simulink model "bit32aluhdl"  (R2020a)
settings: Solver=FixedStepDiscrete  StartTime=0.0  StopTime=10.0  RelTol=1e-3
(part 1 of 66)
settings Model: DataTypeOverride=Off  Creator=kishan  LastModifiedBy=kishan
settings DataIOCC: LimitDataPoints=on  SaveOutput=off  SaveTime=off
settings OptimizationCC: BlockReduction=off  ConditionallyExecuteInputs=off  DefaultParameterBehavior=Inlined  ExpressionDepthLimit=2147483647  InitFltsAndDblsToZero=on  LifeSpan=inf
settings DebuggingCC: AlgebraicLoopMsg=error  UnderspecifiedInitializationDetection=Classic  MergeDetectMultiDrivingBlocksExec=none  SingleTaskRateTransMsg=error  FcnCallInpInsideContextMsg=warning  AllowSymbolicDim=off  StateNameClashWarn=warning  StrictBusMsg=ErrorOnBusTreatedAsVector  SFUnexpectedBacktrackingDiag=warning  SFNoUnconditionalDefaultTransitionDiag=warning  SFExecutionAtInitializationDiag=none  ArithmeticOperatorsInVariantConditions=warning
settings HardwareCC: ProdBitPerPointer=32  ProdBitPerSizeT=32  ProdBitPerPtrDiffT=32  ProdLargestAtomicFloat=None  ProdIntDivRoundTo=Undefined  ProdEndianess=Unspecified  ProdWordSize=32  ProdHWDeviceType=ASIC/FPGA->ASIC/FPGA  ProdEqTarget=off
settings SFSimCC: SimUseLocalCustomCode=off  SimParseCustomCode=off  CustomCodeUndefinedFunction=UseInterfaceOnly
settings RTWCC: RTWUseLocalCustomCode=off
settings CodeAppCC: StateflowObjectComments=on
settings GRTTargetCC: TargetLangStandard=C89/C90 (ANSI)  CombineOutputUpdateFcns=off  GRTInterface=on
settings ConfigComp: CovScope=ReferencedModels  CovMetricSettings=dw  CovHtmlReporting=on  CovSaveCumulativeToWorkspaceVar=on  CovSaveSingleToWorkspaceVar=on  CovExternalEMLEnable=off  CovSFcnEnable=off

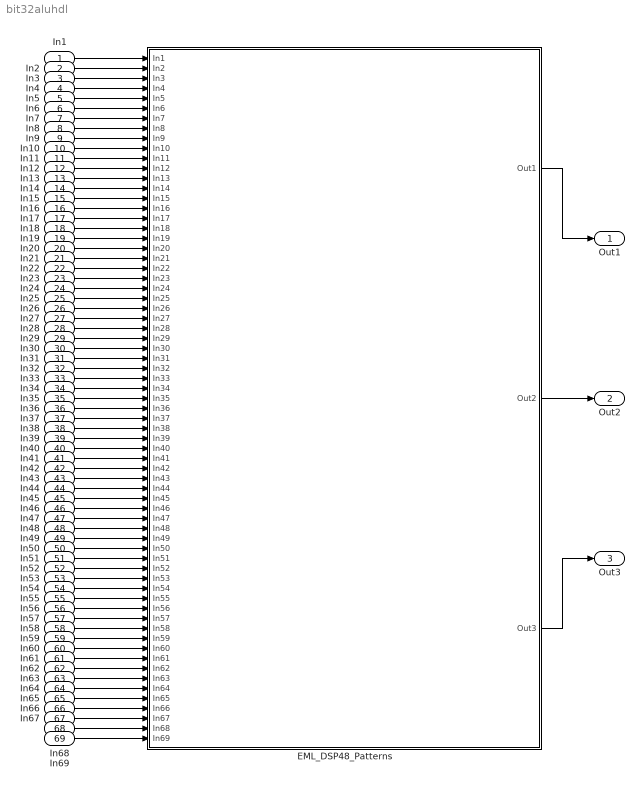
== system bit32aluhdl ==
  In1 : Inport
  In2 : Inport  Port=2
  In3 : Inport  Port=3
  In4 : Inport  Port=4
  In5 : Inport  Port=5
  In6 : Inport  Port=6
  In7 : Inport  Port=7
  In8 : Inport  Port=8
  In9 : Inport  Port=9
  In10 : Inport  Port=10
  In11 : Inport  Port=11
  In12 : Inport  Port=12
  In13 : Inport  Port=13
  In14 : Inport  Port=14
  In15 : Inport  Port=15
  In16 : Inport  Port=16
  In17 : Inport  Port=17
  In18 : Inport  Port=18
  In19 : Inport  Port=19
  In20 : Inport  Port=20
  In21 : Inport  Port=21
  In22 : Inport  Port=22
  In23 : Inport  Port=23
  In24 : Inport  Port=24
  In25 : Inport  Port=25
  In26 : Inport  Port=26
  In27 : Inport  Port=27
  In28 : Inport  Port=28
  In29 : Inport  Port=29
  In30 : Inport  Port=30
  In31 : Inport  Port=31
  In32 : Inport  Port=32
  In33 : Inport  Port=33
  In34 : Inport  Port=34
  In35 : Inport  Port=35
  In36 : Inport  Port=36
  In37 : Inport  Port=37
  In38 : Inport  Port=38
  In39 : Inport  Port=39
  In40 : Inport  Port=40
  In41 : Inport  Port=41
  In42 : Inport  Port=42
  In43 : Inport  Port=43
  In44 : Inport  Port=44
  In45 : Inport  Port=45
  In46 : Inport  Port=46
  In47 : Inport  Port=47
  In48 : Inport  Port=48
  In49 : Inport  Port=49
  In50 : Inport  Port=50
  In51 : Inport  Port=51
  In52 : Inport  Port=52
  In53 : Inport  Port=53
  In54 : Inport  Port=54
  In55 : Inport  Port=55
  In56 : Inport  Port=56
  In57 : Inport  Port=57
  In58 : Inport  Port=58
  In59 : Inport  Port=59
  In60 : Inport  Port=60
  In61 : Inport  Port=61
  In62 : Inport  Port=62
  In63 : Inport  Port=63
  In64 : Inport  Port=64
  In65 : Inport  Port=65
  In66 : Inport  Port=66
  In67 : Inport  Port=67
  In68 : Inport  Port=68
  In69 : Inport  Port=69
  EML_DSP48_Patterns : Subsystem
  Out1 : Outport
  Out2 : Outport  Port=2
  Out3 : Outport  Port=3
  wires:
  EML_DSP48_Patterns/2(Out2) -> Out2/1
  EML_DSP48_Patterns/1(Out1) -> Out1/1
  EML_DSP48_Patterns/3(Out3) -> Out3/1
  In1/1 -> EML_DSP48_Patterns/1(In1)
  In2/1 -> EML_DSP48_Patterns/2(In2)
  In4/1 -> EML_DSP48_Patterns/4(In4)
  In3/1 -> EML_DSP48_Patterns/3(In3)
  In7/1 -> EML_DSP48_Patterns/7(In7)
  In8/1 -> EML_DSP48_Patterns/8(In8)
  In6/1 -> EML_DSP48_Patterns/6(In6)
  In5/1 -> EML_DSP48_Patterns/5(In5)
  In12/1 -> EML_DSP48_Patterns/12(In12)
  In10/1 -> EML_DSP48_Patterns/10(In10)
  In11/1 -> EML_DSP48_Patterns/11(In11)
  In15/1 -> EML_DSP48_Patterns/15(In15)
  In13/1 -> EML_DSP48_Patterns/13(In13)
  In14/1 -> EML_DSP48_Patterns/14(In14)
  In16/1 -> EML_DSP48_Patterns/16(In16)
  In9/1 -> EML_DSP48_Patterns/9(In9)
  In20/1 -> EML_DSP48_Patterns/20(In20)
  In22/1 -> EML_DSP48_Patterns/22(In22)
  In25/1 -> EML_DSP48_Patterns/25(In25)
  In19/1 -> EML_DSP48_Patterns/19(In19)
  In29/1 -> EML_DSP48_Patterns/29(In29)
  In21/1 -> EML_DSP48_Patterns/21(In21)
  In30/1 -> EML_DSP48_Patterns/30(In30)
  In28/1 -> EML_DSP48_Patterns/28(In28)
  In27/1 -> EML_DSP48_Patterns/27(In27)
  In23/1 -> EML_DSP48_Patterns/23(In23)
  In26/1 -> EML_DSP48_Patterns/26(In26)
  In24/1 -> EML_DSP48_Patterns/24(In24)
  In18/1 -> EML_DSP48_Patterns/18(In18)
  In17/1 -> EML_DSP48_Patterns/17(In17)
  In32/1 -> EML_DSP48_Patterns/32(In32)
  In31/1 -> EML_DSP48_Patterns/31(In31)
  In41/1 -> EML_DSP48_Patterns/41(In41)
  In61/1 -> EML_DSP48_Patterns/61(In61)
  In53/1 -> EML_DSP48_Patterns/53(In53)
  In55/1 -> EML_DSP48_Patterns/55(In55)
  In42/1 -> EML_DSP48_Patterns/42(In42)
  In54/1 -> EML_DSP48_Patterns/54(In54)
  In34/1 -> EML_DSP48_Patterns/34(In34)
  In51/1 -> EML_DSP48_Patterns/51(In51)
  In38/1 -> EML_DSP48_Patterns/38(In38)
  In36/1 -> EML_DSP48_Patterns/36(In36)
  In49/1 -> EML_DSP48_Patterns/49(In49)
  In46/1 -> EML_DSP48_Patterns/46(In46)
  In33/1 -> EML_DSP48_Patterns/33(In33)
  In37/1 -> EML_DSP48_Patterns/37(In37)
  In59/1 -> EML_DSP48_Patterns/59(In59)
  In64/1 -> EML_DSP48_Patterns/64(In64)
  In39/1 -> EML_DSP48_Patterns/39(In39)
  In45/1 -> EML_DSP48_Patterns/45(In45)
  In52/1 -> EML_DSP48_Patterns/52(In52)
  In44/1 -> EML_DSP48_Patterns/44(In44)
  In50/1 -> EML_DSP48_Patterns/50(In50)
  In56/1 -> EML_DSP48_Patterns/56(In56)
  In35/1 -> EML_DSP48_Patterns/35(In35)
  In63/1 -> EML_DSP48_Patterns/63(In63)
  In62/1 -> EML_DSP48_Patterns/62(In62)
  In43/1 -> EML_DSP48_Patterns/43(In43)
  In40/1 -> EML_DSP48_Patterns/40(In40)
  In58/1 -> EML_DSP48_Patterns/58(In58)
  In60/1 -> EML_DSP48_Patterns/60(In60)
  In48/1 -> EML_DSP48_Patterns/48(In48)
  In57/1 -> EML_DSP48_Patterns/57(In57)
  In47/1 -> EML_DSP48_Patterns/47(In47)
  In68/1 -> EML_DSP48_Patterns/68(In68)
  In66/1 -> EML_DSP48_Patterns/66(In66)
  In67/1 -> EML_DSP48_Patterns/67(In67)
  In69/1 -> EML_DSP48_Patterns/69(In69)
  In65/1 -> EML_DSP48_Patterns/65(In65)

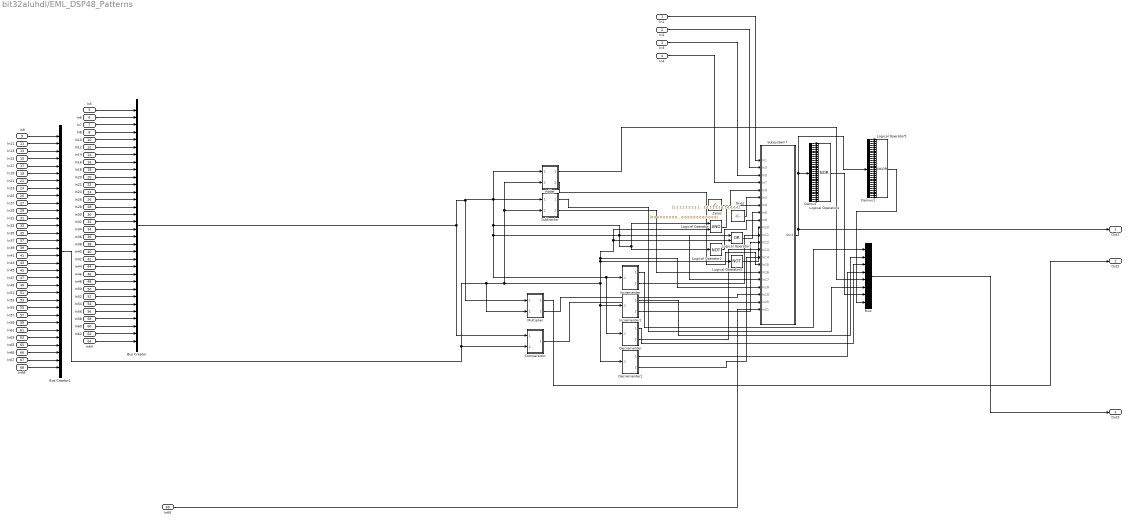
== system bit32aluhdl/EML_DSP48_Patterns ==
  In1 : Inport
  In2 : Inport  Port=2
  In3 : Inport  Port=3
  In4 : Inport  Port=4
  In5 : Inport  Port=5
  In6 : Inport  Port=6
  In7 : Inport  Port=7
  In8 : Inport  Port=8
  In9 : Inport  Port=9
  In10 : Inport  Port=10
  In11 : Inport  Port=11
  In12 : Inport  Port=12
  In13 : Inport  Port=13
  In14 : Inport  Port=14
  In15 : Inport  Port=15
  In16 : Inport  Port=16
  In17 : Inport  Port=17
  In18 : Inport  Port=18
  In19 : Inport  Port=19
  In20 : Inport  Port=20
  In21 : Inport  Port=21
  In22 : Inport  Port=22
  In23 : Inport  Port=23
  In24 : Inport  Port=24
  In25 : Inport  Port=25
  In26 : Inport  Port=26
  In27 : Inport  Port=27
  In28 : Inport  Port=28
  In29 : Inport  Port=29
  In30 : Inport  Port=30
  In31 : Inport  Port=31
  In32 : Inport  Port=32
  In33 : Inport  Port=33
  In34 : Inport  Port=34
  In35 : Inport  Port=35
  In36 : Inport  Port=36
  In37 : Inport  Port=37
  In38 : Inport  Port=38
  In39 : Inport  Port=39
  In40 : Inport  Port=40
  In41 : Inport  Port=41
  In42 : Inport  Port=42
  In43 : Inport  Port=43
  In44 : Inport  Port=44
  In45 : Inport  Port=45
  In46 : Inport  Port=46
  In47 : Inport  Port=47
  In48 : Inport  Port=48
  In49 : Inport  Port=49
  In50 : Inport  Port=50
  In51 : Inport  Port=51
  In52 : Inport  Port=52
  In53 : Inport  Port=53
  In54 : Inport  Port=54
  In55 : Inport  Port=55
  In56 : Inport  Port=56
  In57 : Inport  Port=57
  In58 : Inport  Port=58
  In59 : Inport  Port=59
  In60 : Inport  Port=60
  In61 : Inport  Port=61
  In62 : Inport  Port=62
  In63 : Inport  Port=63
  In64 : Inport  Port=64
  In65 : Inport  Port=65
  In66 : Inport  Port=66
  In67 : Inport  Port=67
  In68 : Inport  Port=68
  In69 : Inport  Port=69
  Adder : Subsystem
  Bus Creator : BusCreator  Inputs=32
  Bus Creator1 : BusCreator  Inputs=32
  Comparartor : Subsystem
  Decrementer : Subsystem
  Decrementer1 : Subsystem
  Demux : Demux  Outputs=32
  Demux1 : Demux  Outputs=32
  Incrementer : Subsystem
  Incrementer1 : Subsystem
  Logical Operator : Logic  AllPortsSameDT=off  OutDataTypeStr=boolean
  Logical Operator1 : Logic  Operator=OR  AllPortsSameDT=off  OutDataTypeStr=boolean
  Logical Operator2 : Logic  Operator=NOT  AllPortsSameDT=off  OutDataTypeStr=boolean
  Logical Operator3 : Logic  Operator=NOT  AllPortsSameDT=off  OutDataTypeStr=boolean
  Logical Operator4 : Logic  Operator=NOR  Inputs=32  AllPortsSameDT=off  OutDataTypeStr=boolean
  Logical Operator5 : Logic  Operator=NXOR  Inputs=32  AllPortsSameDT=off  OutDataTypeStr=boolean
  Multiplier : Subsystem
  Mux : Mux  Inputs=8
  Ones : Constant  Value=[1 1 1 1 1 1 1 1 1 1 1 1 1 1 1 1 1 1 1 1 1 1 1 1 1 1 1 1 1 1 1 1]  OutDataTypeStr=boolean
  Subsystem7 : Subsystem
  Subtractor : Subsystem
  Zeros : Constant  Value=[0 0 0 0 0 0 0 0 0 0 0 0 0 0 0 0 0 0 0 0 0 0 0 0 0 0 0 0 0 0 0 0]  OutDataTypeStr=boolean
  Out1 : Outport
  Out2 : Outport  Port=2
  Out3 : Outport  Port=3
  wires:
  Mux/1 -> Out3/1
  In68/1 -> Bus Creator1/32
  In65/1 -> Bus Creator1/29
  In62/1 -> Bus Creator/31
  In55/1 -> Bus Creator1/24
  Demux/2 -> Logical Operator4/2
  In53/1 -> Bus Creator1/23
  In51/1 -> Bus Creator1/22
  Adder/2(Out2) -> Subsystem7/15(In15)
  In50/1 -> Bus Creator/25
  In47/1 -> Bus Creator1/20
  In43/1 -> Bus Creator1/18
  In41/1 -> Bus Creator1/17
  Multiplier/1(Out1) -> Out2/1
  Incrementer1/1(Out1) -> Mux/2
  In48/1 -> Bus Creator/24
  In38/1 -> Bus Creator/19
  In61/1 -> Bus Creator1/27
  In37/1 -> Bus Creator1/15
  In46/1 -> Bus Creator/23
  In36/1 -> Bus Creator/18
  Demux/30 -> Logical Operator4/30
  Demux/27 -> Logical Operator4/27
  In34/1 -> Bus Creator/17
  Demux/32 -> Logical Operator4/32
  In33/1 -> Bus Creator1/13
  In23/1 -> Bus Creator1/8
  In30/1 -> Bus Creator/15
  In29/1 -> Bus Creator1/11
  Demux/5 -> Logical Operator4/5
  In28/1 -> Bus Creator/14
  In3/1 -> Subsystem7/3(In5)
  In26/1 -> Bus Creator/13
  Demux1/14 -> Logical Operator5/14
  In42/1 -> Bus Creator/21
  In24/1 -> Bus Creator/12
  In22/1 -> Bus Creator/11
  In32/1 -> Bus Creator/16
  In16/1 -> Bus Creator/8
  In20/1 -> Bus Creator/10
  In18/1 -> Bus Creator/9
  In14/1 -> Bus Creator/7
  In58/1 -> Bus Creator/29
  In13/1 -> Bus Creator1/3
  In57/1 -> Bus Creator1/25
  In12/1 -> Bus Creator/6
  In9/1 -> Bus Creator1/1
  In8/1 -> Bus Creator/4
  In7/1 -> Bus Creator/3
  Bus Creator1/1 -> Subsystem7/18(In18), Logical Operator1/2, Logical Operator/2, Logical Operator3/1, Incrementer1/1(In1), Decrementer1/1(In1), Subtractor/2(In2), Adder/2(In2), Multiplier/2(In2), Comparartor/2(In2)
  In21/1 -> Bus Creator1/7
  In4/1 -> Subsystem7/4(In7)
  In2/1 -> Subsystem7/2(In3)
  In60/1 -> Bus Creator/30
  Zeros/1 -> Subsystem7/5(In9)
  Ones/1 -> Subsystem7/6(In2)
  Demux/31 -> Logical Operator4/31
  In17/1 -> Bus Creator1/5
  Logical Operator2/1 -> Subsystem7/9(In8)
  Logical Operator/1 -> Subsystem7/7(In4)
  Demux1/8 -> Logical Operator5/8
  Demux/11 -> Logical Operator4/11
  Logical Operator5/1 -> Mux/8
  Demux/29 -> Logical Operator4/29
  In10/1 -> Bus Creator/5
  In40/1 -> Bus Creator/20
  Decrementer1/1(Out1) -> Mux/4
  Demux/19 -> Logical Operator4/19
  Demux1/3 -> Logical Operator5/3
  Incrementer/1(Out1) -> Mux/1
  Demux/13 -> Logical Operator4/13
  Demux1/20 -> Logical Operator5/20
  Demux/24 -> Logical Operator4/24
  In5/1 -> Bus Creator/1
  Demux1/10 -> Logical Operator5/10
  Demux1/2 -> Logical Operator5/2
  Decrementer1/2(Out2) -> Subsystem7/14(In14)
  Demux1/21 -> Logical Operator5/21
  Demux/7 -> Logical Operator4/7
  In25/1 -> Bus Creator1/9
  Demux1/25 -> Logical Operator5/25
  Demux/15 -> Logical Operator4/15
  Demux/25 -> Logical Operator4/25
  Demux1/1 -> Logical Operator5/1
  In54/1 -> Bus Creator/27
  Demux/26 -> Logical Operator4/26
  Demux1/22 -> Logical Operator5/22
  Demux/17 -> Logical Operator4/17
  In56/1 -> Bus Creator/28
  Logical Operator1/1 -> Subsystem7/8(In6)
  Demux1/4 -> Logical Operator5/4
  Demux1/6 -> Logical Operator5/6
  In45/1 -> Bus Creator1/19
  Demux/4 -> Logical Operator4/4
  In35/1 -> Bus Creator1/14
  Demux1/7 -> Logical Operator5/7
  In31/1 -> Bus Creator1/12
  In15/1 -> Bus Creator1/4
  Demux1/30 -> Logical Operator5/30
  In11/1 -> Bus Creator1/2
  Subsystem7/1(Out1) -> Out1/1, Demux1/1, Demux/1
  In63/1 -> Bus Creator1/28
  In64/1 -> Bus Creator/32
  Demux/16 -> Logical Operator4/16
  Demux1/15 -> Logical Operator5/15
  Demux/18 -> Logical Operator4/18
  In69/1 -> Subsystem7/21(In21)
  Demux1/26 -> Logical Operator5/26
  Adder/1(Out1) -> Mux/5
  In27/1 -> Bus Creator1/10
  Demux1/18 -> Logical Operator5/18
  Demux1/29 -> Logical Operator5/29
  Incrementer1/2(Out2) -> Subsystem7/12(In12)
  Subtractor/2(Out2) -> Subsystem7/16(In16)
  Demux/9 -> Logical Operator4/9
  Logical Operator4/1 -> Mux/7
  Demux1/16 -> Logical Operator5/16
  Demux/20 -> Logical Operator4/20
  In49/1 -> Bus Creator1/21
  In39/1 -> Bus Creator1/16
  Demux/21 -> Logical Operator4/21
  Demux1/24 -> Logical Operator5/24
  Demux1/9 -> Logical Operator5/9
  Demux/8 -> Logical Operator4/8
  In59/1 -> Bus Creator1/26
  Demux1/19 -> Logical Operator5/19
  In67/1 -> Bus Creator1/31
  Demux1/32 -> Logical Operator5/32
  In52/1 -> Bus Creator/26
  Demux/10 -> Logical Operator4/10
  In44/1 -> Bus Creator/22
  In66/1 -> Bus Creator1/30
  Demux1/23 -> Logical Operator5/23
  Decrementer/2(Out2) -> Subsystem7/13(In13)
  Demux/6 -> Logical Operator4/6
  Subtractor/1(Out1) -> Mux/6
  Demux/28 -> Logical Operator4/28
  In19/1 -> Bus Creator1/6
  Demux1/13 -> Logical Operator5/13
  Demux1/12 -> Logical Operator5/12
  Demux1/11 -> Logical Operator5/11
  In1/1 -> Subsystem7/1(In1)
  Bus Creator/1 -> Adder/1(In1), Subsystem7/17(In17), Decrementer/1(In1), Incrementer/1(In1), Logical Operator2/1, Logical Operator/1, Logical Operator1/1, Subtractor/1(In1), Multiplier/1(In1), Comparartor/1(In1)
  Demux1/5 -> Logical Operator5/5
  Demux/14 -> Logical Operator4/14
  Logical Operator3/1 -> Subsystem7/10(In10)
  Demux1/17 -> Logical Operator5/17
  Decrementer/1(Out1) -> Mux/3
  Demux1/27 -> Logical Operator5/27
  In6/1 -> Bus Creator/2
  Demux/3 -> Logical Operator4/3
  Demux/1 -> Logical Operator4/1
  Demux/12 -> Logical Operator4/12
  Demux/23 -> Logical Operator4/23
  Demux1/31 -> Logical Operator5/31
  Incrementer/2(Out2) -> Subsystem7/11(In11)
  Demux1/28 -> Logical Operator5/28
  Multiplier/2(Out2) -> Subsystem7/19(In19)
  Comparartor/1(Out1) -> Subsystem7/20(In20)
  Demux/22 -> Logical Operator4/22

== system bit32aluhdl/EML_DSP48_Patterns/Adder ==
  In1 : Inport
  In2 : Inport  Port=2
  Subsystem : Subsystem
  Zeros1 : Constant  Value=0  OutDataTypeStr=boolean
  Out1 : Outport
  Out2 : Outport  Port=2
  wires:
  Subsystem/2(Out2) -> Out2/1
  In2/1 -> Subsystem/3(In3)
  Zeros1/1 -> Subsystem/2(In2)
  In1/1 -> Subsystem/1(In1)
  Subsystem/1(Out1) -> Out1/1

== system bit32aluhdl/EML_DSP48_Patterns/Comparartor ==
  In1 : Inport
  In2 : Inport  Port=2
  Comparator : Subsystem
  Comparator1 : Subsystem
  Comparator2 : Subsystem
  Comparator3 : Subsystem
  Demux : Demux
  Demux1 : Demux
  Display : Display
  Logical Operator : Logic  Operator=OR  Inputs=4  AllPortsSameDT=off  OutDataTypeStr=boolean
  Logical Operator1 : Logic  Inputs=4  AllPortsSameDT=off  OutDataTypeStr=boolean
  Logical Operator2 : Logic  AllPortsSameDT=off  OutDataTypeStr=boolean
  Logical Operator3 : Logic  Inputs=3  AllPortsSameDT=off  OutDataTypeStr=boolean
  Logical Operator4 : Logic  Inputs=4  AllPortsSameDT=off  OutDataTypeStr=boolean
  Logical Operator5 : Logic  Operator=NOR  AllPortsSameDT=off  OutDataTypeStr=boolean
  Mux : Mux
  Mux1 : Mux
  Zeros1 : Constant  Value=[0 0 0 0 0 0 0 0 0 0 0 0 0 0 0 0 0 0 0 0 0 0 0 0 0 0 0 0 0]  OutDataTypeStr=boolean
  Out1 : Outport
  wires:
  Zeros1/1 -> Mux/4
  Mux/1 -> Out1/1
  In1/1 -> Demux/1
  In2/1 -> Demux1/1
  Demux/1 -> Comparator/1(In1)
  Demux/2 -> Comparator1/1(In1)
  Demux/3 -> Comparator2/1(In1)
  Demux/4 -> Comparator3/1(In1)
  Demux1/1 -> Comparator/2(In2)
  Demux1/2 -> Comparator1/2(In2)
  Demux1/3 -> Comparator2/2(In2)
  Demux1/4 -> Comparator3/2(In2)
  Comparator/2(Out2) -> Logical Operator1/1, Logical Operator4/1, Logical Operator3/1, Logical Operator2/1
  Comparator1/2(Out2) -> Logical Operator4/2, Logical Operator3/2, Logical Operator1/2
  Comparator2/2(Out2) -> Logical Operator4/3, Logical Operator1/3
  Comparator3/2(Out2) -> Logical Operator1/4
  Logical Operator1/1 -> Logical Operator5/2, Mux/2
  Mux1/1 -> Display/1
  Comparator/1(Out1) -> Logical Operator/1
  Comparator1/1(Out1) -> Logical Operator2/2
  Logical Operator2/1 -> Logical Operator/2
  Comparator2/1(Out1) -> Logical Operator3/3
  Logical Operator3/1 -> Logical Operator/3
  Comparator3/1(Out1) -> Logical Operator4/4
  Logical Operator4/1 -> Logical Operator/4
  Logical Operator/1 -> Logical Operator5/1, Mux/1
  Comparator/3(Out3) -> Mux1/1
  Comparator1/3(Out3) -> Mux1/2
  Comparator2/3(Out3) -> Mux1/3
  Comparator3/3(Out3) -> Mux1/4
  Logical Operator5/1 -> Mux/3

== system bit32aluhdl/EML_DSP48_Patterns/Decrementer ==
  In1 : Inport
  Subtractor1 : Subsystem
  Zeros1 : Constant  Value=[0 0 0 0 0 0 0 0 0 0 0 0 0 0 0 0 0 0 0 0 0 0 0 0 0 0 0 0 0 0 0 1]
  Out1 : Outport
  Out2 : Outport  Port=2
  wires:
  Zeros1/1 -> Subtractor1/2(In2)
  In1/1 -> Subtractor1/1(In1)
  Subtractor1/1(Out1) -> Out1/1
  Subtractor1/2(Out2) -> Out2/1

== system bit32aluhdl/EML_DSP48_Patterns/Decrementer1 ==
  In1 : Inport
  Subtractor1 : Subsystem
  Zeros1 : Constant  Value=[0 0 0 0 0 0 0 0 0 0 0 0 0 0 0 0 0 0 0 0 0 0 0 0 0 0 0 0 0 0 0 1]
  Out1 : Outport
  Out2 : Outport  Port=2
  wires:
  Zeros1/1 -> Subtractor1/2(In2)
  In1/1 -> Subtractor1/1(In1)
  Subtractor1/1(Out1) -> Out1/1
  Subtractor1/2(Out2) -> Out2/1

== system bit32aluhdl/EML_DSP48_Patterns/Incrementer ==
  In1 : Inport
  Incrementer : Subsystem
  Zeros1 : Constant  Value=[0 0 0 0 0 0 0 0 0 0 0 0 0 0 0 0 0 0 0 0 0 0 0 0 0 0 0 0 0 0 0 1]  OutDataTypeStr=boolean
  Out1 : Outport
  Out2 : Outport  Port=2
  wires:
  Zeros1/1 -> Incrementer/2(In2)
  In1/1 -> Incrementer/1(In1)
  Incrementer/2(Out2) -> Out2/1
  Incrementer/1(Out1) -> Out1/1

== system bit32aluhdl/EML_DSP48_Patterns/Incrementer1 ==
  In1 : Inport
  Incrementer : Subsystem
  Zeros1 : Constant  Value=[0 0 0 0 0 0 0 0 0 0 0 0 0 0 0 0 0 0 0 0 0 0 0 0 0 0 0 0 0 0 0 1]  OutDataTypeStr=boolean
  Out1 : Outport
  Out2 : Outport  Port=2
  wires:
  Zeros1/1 -> Incrementer/2(In2)
  In1/1 -> Incrementer/1(In1)
  Incrementer/2(Out2) -> Out2/1
  Incrementer/1(Out1) -> Out1/1

== system bit32aluhdl/EML_DSP48_Patterns/Multiplier ==
  In1 : Inport
  In2 : Inport  Port=2
  Constant : Constant  Value=0  OutDataTypeStr=boolean
  Constant1 : Constant  Value=0  OutDataTypeStr=boolean
  Constant2 : Constant  Value=[0 0 0 0 0 0 0 0 0 0 0 0 0 0 0]  OutDataTypeStr=boolean
  Demux : Demux  Outputs=2
  Demux1 : Demux  Outputs=2
  Demux2 : Demux  Outputs=2
  Display : Display
  Logical Operator : Logic  AllPortsSameDT=off  OutDataTypeStr=boolean
  Logical Operator1 : Logic  Operator=XOR  AllPortsSameDT=off  OutDataTypeStr=boolean
  Mux{,1..3} (4 alike) : Mux  Inputs=2
  Mux4 : Mux  Inputs=3
  Subsystem : Subsystem
  Subsystem1 : Subsystem
  Subsystem2 : Subsystem
  Subsystem3 : Subsystem
  Subsystem4 : Subsystem
  Subsystem5 : Subsystem
  Subsystem7 : Subsystem
  Out1 : Outport
  Out2 : Outport  Port=2
  wires:
  Constant1/1 -> Subsystem4/2(In2)
  Subsystem3/1(Out1) -> Mux2/2
  Logical Operator/1 -> Subsystem5/2(In2)
  Subsystem3/2(Out2) -> Mux4/3
  Subsystem5/2(Out2) -> Mux4/1
  Demux/2 -> Subsystem3/1(In1), Subsystem2/1(In1)
  Mux1/1 -> Subsystem/3(In3)
  Mux3/1 -> Subsystem5/3(In3)
  Subsystem4/1(Out1) -> Logical Operator/2, Logical Operator1/2
  Logical Operator1/1 -> Mux3/2
  Subsystem2/1(Out1) -> Mux1/1
  Subsystem/1(Out1) -> Logical Operator/1, Logical Operator1/1
  Subsystem5/1(Out1) -> Display/1
  In1/1 -> Demux/1
  Demux1/2 -> Subsystem1/2(In2), Subsystem3/2(In2)
  Constant/1 -> Subsystem/2(In2)
  Subsystem7/1(Out1) -> Subsystem5/1(In1)
  In2/1 -> Demux1/1
  Subsystem7/2(Out2) -> Mux2/1
  Subsystem4/2(Out2) -> Mux4/2
  Subsystem/2(Out2) -> Subsystem4/1(In1)
  Demux/1 -> Subsystem1/1(In1), Subsystem7/1(In1)
  Subsystem1/2(Out2) -> Mux/2
  Demux1/1 -> Subsystem7/2(In2), Subsystem2/2(In2)
  Constant2/1 -> Mux3/1
  Subsystem2/2(Out2) -> Mux1/2
  Mux/1 -> Subsystem/1(In1)
  Mux2/1 -> Subsystem4/3(In3)
  Subsystem1/1(Out1) -> Mux/1
  Mux4/1 -> Demux2/1
  Demux2/1 -> Out1/1
  Demux2/2 -> Out2/1

== system bit32aluhdl/EML_DSP48_Patterns/Subsystem7 ==
  In1 : Inport
  In3 : Inport  Port=2
  In5 : Inport  Port=3
  In7 : Inport  Port=4
  In9 : Inport  Port=5
  In2 : Inport  Port=6
  In4 : Inport  Port=7
  In6 : Inport  Port=8
  In8 : Inport  Port=9
  In10 : Inport  Port=10
  In11 : Inport  Port=11
  In12 : Inport  Port=12
  In13 : Inport  Port=13
  In14 : Inport  Port=14
  In15 : Inport  Port=15
  In16 : Inport  Port=16
  In17 : Inport  Port=17
  In18 : Inport  Port=18
  In19 : Inport  Port=19
  In20 : Inport  Port=20
  In21 : Inport  Port=21
  Demux{,1..15} (16 alike) : Demux
  Mux : Mux
  Subsystem1 : Subsystem
  Subsystem2 : Subsystem
  Subsystem3 : Subsystem
  Subsystem4 : Subsystem
  Out1 : Outport
  wires:
  In3/1 -> Subsystem3/2(In21), Subsystem4/2(In21), Subsystem2/2(In21), Subsystem1/2(In21)
  In7/1 -> Subsystem4/4(In2), Subsystem3/4(In2), Subsystem2/4(In2), Subsystem1/4(In2)
  Subsystem3/1(Out1) -> Mux/1
  Subsystem4/1(Out1) -> Mux/2
  Subsystem2/1(Out1) -> Mux/4
  In5/1 -> Subsystem4/3(In1), Subsystem3/3(In1), Subsystem2/3(In1), Subsystem1/3(In1)
  In1/1 -> Subsystem4/1(In20), Subsystem3/1(In20), Subsystem2/1(In20), Subsystem1/1(In20)
  Subsystem1/1(Out1) -> Mux/3
  Mux/1 -> Out1/1
  In9/1 -> Demux/1
  In21/1 -> Subsystem4/21(In19), Subsystem3/21(In19), Subsystem2/21(In19), Subsystem1/21(In19)
  Demux/1 -> Subsystem3/5(In3)
  Demux/2 -> Subsystem4/5(In3)
  Demux/3 -> Subsystem1/5(In3)
  Demux/4 -> Subsystem2/5(In3)
  Demux1/4 -> Subsystem2/6(In4)
  Demux1/1 -> Subsystem3/6(In4)
  Demux1/2 -> Subsystem4/6(In4)
  Demux1/3 -> Subsystem1/6(In4)
  In2/1 -> Demux1/1
  Demux2/2 -> Subsystem4/7(In5)
  Demux3/1 -> Subsystem3/8(In6)
  Demux2/3 -> Subsystem1/7(In5)
  Demux3/2 -> Subsystem4/8(In6)
  Demux2/4 -> Subsystem2/7(In5)
  In6/1 -> Demux3/1
  Demux2/1 -> Subsystem3/7(In5)
  Demux3/3 -> Subsystem1/8(In6)
  Demux3/4 -> Subsystem2/8(In6)
  In4/1 -> Demux2/1
  In10/1 -> Demux5/1
  In11/1 -> Demux6/1
  Demux6/3 -> Subsystem1/11(In9)
  Demux4/2 -> Subsystem4/9(In7)
  Demux7/2 -> Subsystem4/12(In10)
  Demux5/1 -> Subsystem3/10(In8)
  Demux5/2 -> Subsystem4/10(In8)
  Demux4/3 -> Subsystem1/9(In7)
  Demux4/4 -> Subsystem2/9(In7)
  Demux6/4 -> Subsystem2/11(In9)
  Demux7/1 -> Subsystem3/12(In10)
  Demux6/2 -> Subsystem4/11(In9)
  Demux7/4 -> Subsystem2/12(In10)
  Demux4/1 -> Subsystem3/9(In7)
  Demux6/1 -> Subsystem3/11(In9)
  Demux5/4 -> Subsystem2/10(In8)
  Demux5/3 -> Subsystem1/10(In8)
  Demux7/3 -> Subsystem1/12(In10)
  In12/1 -> Demux7/1
  In8/1 -> Demux4/1
  Demux11/4 -> Subsystem2/16(In14)
  Demux15/1 -> Subsystem3/20(In18)
  Demux10/2 -> Subsystem4/15(In13)
  In20/1 -> Demux15/1
  Demux8/2 -> Subsystem4/13(In11)
  Demux12/4 -> Subsystem2/17(In15)
  Demux13/1 -> Subsystem3/18(In16)
  Demux13/4 -> Subsystem2/18(In16)
  Demux11/3 -> Subsystem1/16(In14)
  Demux15/4 -> Subsystem2/20(In18)
  Demux10/4 -> Subsystem2/15(In13)
  Demux15/3 -> Subsystem1/20(In18)
  In14/1 -> Demux9/1
  Demux9/4 -> Subsystem2/14(In12)
  Demux14/4 -> Subsystem2/19(In17)
  Demux12/2 -> Subsystem4/17(In15)
  Demux8/3 -> Subsystem1/13(In11)
  Demux15/2 -> Subsystem4/20(In18)
  Demux9/2 -> Subsystem4/14(In12)
  In15/1 -> Demux10/1
  Demux11/2 -> Subsystem4/16(In14)
  Demux14/1 -> Subsystem3/19(In17)
  Demux12/1 -> Subsystem3/17(In15)
  Demux10/3 -> Subsystem1/15(In13)
  Demux12/3 -> Subsystem1/17(In15)
  Demux13/2 -> Subsystem4/18(In16)
  Demux9/1 -> Subsystem3/14(In12)
  Demux11/1 -> Subsystem3/16(In14)
  Demux8/1 -> Subsystem3/13(In11)
  Demux14/3 -> Subsystem1/19(In17)
  Demux14/2 -> Subsystem4/19(In17)
  Demux13/3 -> Subsystem1/18(In16)
  Demux8/4 -> Subsystem2/13(In11)
  Demux10/1 -> Subsystem3/15(In13)
  In19/1 -> Demux14/1
  Demux9/3 -> Subsystem1/14(In12)
  In18/1 -> Demux13/1
  In16/1 -> Demux11/1
  In17/1 -> Demux12/1
  In13/1 -> Demux8/1

== system bit32aluhdl/EML_DSP48_Patterns/Subtractor ==
  In1 : Inport
  In2 : Inport  Port=2
  Logical Operator2 : Logic  Operator=NOT  AllPortsSameDT=off  OutDataTypeStr=boolean
  Subtractor : Subsystem
  Zeros1 : Constant  OutDataTypeStr=boolean
  Out1 : Outport
  Out2 : Outport  Port=2
  wires:
  In2/1 -> Logical Operator2/1
  Subtractor/1(Out1) -> Out1/1
  In1/1 -> Subtractor/1(In1)
  Subtractor/2(Out2) -> Out2/1
  Logical Operator2/1 -> Subtractor/3(In3)
  Zeros1/1 -> Subtractor/2(In2)

== system bit32aluhdl/EML_DSP48_Patterns/Adder/Subsystem ==
  In1 : Inport
  In2 : Inport  Port=2
  In3 : Inport  Port=3
  Demux : Demux  Outputs=2
  Demux1 : Demux  Outputs=2
  Mux : Mux  Inputs=2
  Subsystem1 : Subsystem
  Subsystem2 : Subsystem
  Out1 : Outport
  Out2 : Outport  Port=2
  wires:
  Mux/1 -> Out2/1
  In3/1 -> Demux1/1
  Subsystem2/2(Out2) -> Mux/2
  In1/1 -> Demux/1
  Subsystem2/1(Out1) -> Subsystem1/2(In2)
  Subsystem1/2(Out2) -> Mux/1
  Demux1/2 -> Subsystem2/3(In3)
  In2/1 -> Subsystem2/2(In2)
  Demux/2 -> Subsystem2/1(In1)
  Subsystem1/1(Out1) -> Out1/1
  Demux1/1 -> Subsystem1/3(In3)
  Demux/1 -> Subsystem1/1(In1)

== system bit32aluhdl/EML_DSP48_Patterns/Comparartor/Comparator ==
  In1 : Inport
  In2 : Inport  Port=2
  Demux{,1..3} (4 alike) : Demux  Outputs=8
  Logical Operator{1..3,7,9..12,14..15,17..18,21,23..24} (15 alike) : Logic  Operator=NOT  Inputs=3  AllPortsSameDT=off  OutDataTypeStr=boolean
  Logical Operator{4,8,13,16,19..20,22} (7 alike) : Logic  Inputs=3  AllPortsSameDT=off  OutDataTypeStr=boolean
  Logical Operator25 : Logic  Operator=NOR  AllPortsSameDT=off  OutDataTypeStr=boolean
  Logical Operator5 : Logic  AllPortsSameDT=off  OutDataTypeStr=boolean
  Logical Operator6 : Logic  Operator=OR  Inputs=8  AllPortsSameDT=off  OutDataTypeStr=boolean
  NOT{1..8} (8 alike) : Logic  Operator=NXOR  AllPortsSameDT=off  OutDataTypeStr=boolean
  NOT9 : Logic  Inputs=8  AllPortsSameDT=off  OutDataTypeStr=boolean
  Out1 : Outport
  Out2 : Outport  Port=2
  Out3 : Outport  Port=3
  wires:
  Demux/1 -> NOT1/1
  Demux/2 -> NOT2/1
  Demux/3 -> NOT3/1
  Demux/4 -> NOT4/1
  Demux/5 -> NOT5/1
  Demux/6 -> NOT6/1
  Demux/7 -> NOT7/1
  Demux/8 -> NOT8/1
  Demux1/1 -> NOT1/2
  Demux1/2 -> NOT2/2
  Demux1/3 -> NOT3/2
  Demux1/4 -> NOT4/2
  Demux1/5 -> NOT5/2
  Demux1/6 -> NOT6/2
  Demux1/7 -> NOT7/2
  Demux1/8 -> NOT8/2
  In1/1 -> Demux2/1, Demux/1
  In2/1 -> Demux1/1, Demux3/1
  NOT1/1 -> NOT9/1
  NOT2/1 -> NOT9/2
  NOT3/1 -> NOT9/3
  NOT4/1 -> NOT9/4
  NOT5/1 -> NOT9/5
  NOT6/1 -> NOT9/6
  NOT7/1 -> NOT9/7
  NOT8/1 -> NOT9/8
  NOT9/1 -> Logical Operator25/2, Out2/1
  Logical Operator14/1 -> Logical Operator16/3
  Logical Operator7/1 -> Logical Operator8/1
  Logical Operator13/1 -> Logical Operator15/1, Logical Operator6/3
  Demux3/1 -> Logical Operator9/1
  Demux2/2 -> Logical Operator8/2
  Logical Operator15/1 -> Logical Operator16/1
  Demux2/3 -> Logical Operator13/2
  Logical Operator10/1 -> Logical Operator8/3
  Logical Operator6/1 -> Logical Operator25/1, Out1/1
  Demux2/1 -> Logical Operator5/1
  Demux2/4 -> Logical Operator16/2
  Logical Operator11/1 -> Logical Operator13/3
  Logical Operator16/1 -> Logical Operator24/1, Logical Operator6/4
  Logical Operator9/1 -> Logical Operator5/2
  Demux3/2 -> Logical Operator10/1
  Logical Operator12/1 -> Logical Operator13/1
  Demux3/3 -> Logical Operator11/1
  Demux3/4 -> Logical Operator14/1
  Logical Operator5/1 -> Logical Operator7/1, Logical Operator6/1
  Logical Operator8/1 -> Logical Operator12/1, Logical Operator6/2
  Demux2/5 -> Logical Operator20/1
  Demux3/5 -> Logical Operator23/1
  Logical Operator17/1 -> Logical Operator19/3
  Logical Operator19/1 -> Logical Operator6/8
  Logical Operator1/1 -> Logical Operator22/3
  Logical Operator2/1 -> Logical Operator4/3
  Demux3/8 -> Logical Operator17/1
  Demux3/7 -> Logical Operator2/1
  Demux2/7 -> Logical Operator4/2
  Logical Operator3/1 -> Logical Operator4/1
  Logical Operator21/1 -> Logical Operator22/1
  Logical Operator22/1 -> Logical Operator6/6, Logical Operator3/1
  Demux2/8 -> Logical Operator19/2
  Logical Operator18/1 -> Logical Operator19/1
  Logical Operator20/1 -> Logical Operator6/5, Logical Operator21/1
  Demux3/6 -> Logical Operator1/1
  Logical Operator4/1 -> Logical Operator6/7, Logical Operator18/1
  Demux2/6 -> Logical Operator22/2
  Logical Operator24/1 -> Logical Operator20/2
  Logical Operator23/1 -> Logical Operator20/3
  Logical Operator25/1 -> Out3/1

== system bit32aluhdl/EML_DSP48_Patterns/Comparartor/Comparator1 ==
  In1 : Inport
  In2 : Inport  Port=2
  Demux{,1..3} (4 alike) : Demux  Outputs=8
  Logical Operator{1..3,7,9..12,14..15,17..18,21,23..24} (15 alike) : Logic  Operator=NOT  Inputs=3  AllPortsSameDT=off  OutDataTypeStr=boolean
  Logical Operator{4,8,13,16,19..20,22} (7 alike) : Logic  Inputs=3  AllPortsSameDT=off  OutDataTypeStr=boolean
  Logical Operator25 : Logic  Operator=NOR  AllPortsSameDT=off  OutDataTypeStr=boolean
  Logical Operator5 : Logic  AllPortsSameDT=off  OutDataTypeStr=boolean
  Logical Operator6 : Logic  Operator=OR  Inputs=8  AllPortsSameDT=off  OutDataTypeStr=boolean
  NOT{1..8} (8 alike) : Logic  Operator=NXOR  AllPortsSameDT=off  OutDataTypeStr=boolean
  NOT9 : Logic  Inputs=8  AllPortsSameDT=off  OutDataTypeStr=boolean
  Out1 : Outport
  Out2 : Outport  Port=2
  Out3 : Outport  Port=3
  wires:
  Demux/1 -> NOT1/1
  Demux/2 -> NOT2/1
  Demux/3 -> NOT3/1
  Demux/4 -> NOT4/1
  Demux/5 -> NOT5/1
  Demux/6 -> NOT6/1
  Demux/7 -> NOT7/1
  Demux/8 -> NOT8/1
  Demux1/1 -> NOT1/2
  Demux1/2 -> NOT2/2
  Demux1/3 -> NOT3/2
  Demux1/4 -> NOT4/2
  Demux1/5 -> NOT5/2
  Demux1/6 -> NOT6/2
  Demux1/7 -> NOT7/2
  Demux1/8 -> NOT8/2
  In1/1 -> Demux2/1, Demux/1
  In2/1 -> Demux1/1, Demux3/1
  NOT1/1 -> NOT9/1
  NOT2/1 -> NOT9/2
  NOT3/1 -> NOT9/3
  NOT4/1 -> NOT9/4
  NOT5/1 -> NOT9/5
  NOT6/1 -> NOT9/6
  NOT7/1 -> NOT9/7
  NOT8/1 -> NOT9/8
  NOT9/1 -> Logical Operator25/2, Out2/1
  Logical Operator14/1 -> Logical Operator16/3
  Logical Operator7/1 -> Logical Operator8/1
  Logical Operator13/1 -> Logical Operator15/1, Logical Operator6/3
  Demux3/1 -> Logical Operator9/1
  Demux2/2 -> Logical Operator8/2
  Logical Operator15/1 -> Logical Operator16/1
  Demux2/3 -> Logical Operator13/2
  Logical Operator10/1 -> Logical Operator8/3
  Logical Operator6/1 -> Logical Operator25/1, Out1/1
  Demux2/1 -> Logical Operator5/1
  Demux2/4 -> Logical Operator16/2
  Logical Operator11/1 -> Logical Operator13/3
  Logical Operator16/1 -> Logical Operator24/1, Logical Operator6/4
  Logical Operator9/1 -> Logical Operator5/2
  Demux3/2 -> Logical Operator10/1
  Logical Operator12/1 -> Logical Operator13/1
  Demux3/3 -> Logical Operator11/1
  Demux3/4 -> Logical Operator14/1
  Logical Operator5/1 -> Logical Operator7/1, Logical Operator6/1
  Logical Operator8/1 -> Logical Operator12/1, Logical Operator6/2
  Demux2/5 -> Logical Operator20/1
  Demux3/5 -> Logical Operator23/1
  Logical Operator17/1 -> Logical Operator19/3
  Logical Operator19/1 -> Logical Operator6/8
  Logical Operator1/1 -> Logical Operator22/3
  Logical Operator2/1 -> Logical Operator4/3
  Demux3/8 -> Logical Operator17/1
  Demux3/7 -> Logical Operator2/1
  Demux2/7 -> Logical Operator4/2
  Logical Operator3/1 -> Logical Operator4/1
  Logical Operator21/1 -> Logical Operator22/1
  Logical Operator22/1 -> Logical Operator6/6, Logical Operator3/1
  Demux2/8 -> Logical Operator19/2
  Logical Operator18/1 -> Logical Operator19/1
  Logical Operator20/1 -> Logical Operator6/5, Logical Operator21/1
  Demux3/6 -> Logical Operator1/1
  Logical Operator4/1 -> Logical Operator6/7, Logical Operator18/1
  Demux2/6 -> Logical Operator22/2
  Logical Operator24/1 -> Logical Operator20/2
  Logical Operator23/1 -> Logical Operator20/3
  Logical Operator25/1 -> Out3/1

== system bit32aluhdl/EML_DSP48_Patterns/Comparartor/Comparator2 ==
  In1 : Inport
  In2 : Inport  Port=2
  Demux{,1..3} (4 alike) : Demux  Outputs=8
  Logical Operator{1..3,7,9..12,14..15,17..18,21,23..24} (15 alike) : Logic  Operator=NOT  Inputs=3  AllPortsSameDT=off  OutDataTypeStr=boolean
  Logical Operator{4,8,13,16,19..20,22} (7 alike) : Logic  Inputs=3  AllPortsSameDT=off  OutDataTypeStr=boolean
  Logical Operator25 : Logic  Operator=NOR  AllPortsSameDT=off  OutDataTypeStr=boolean
  Logical Operator5 : Logic  AllPortsSameDT=off  OutDataTypeStr=boolean
  Logical Operator6 : Logic  Operator=OR  Inputs=8  AllPortsSameDT=off  OutDataTypeStr=boolean
  NOT{1..8} (8 alike) : Logic  Operator=NXOR  AllPortsSameDT=off  OutDataTypeStr=boolean
  NOT9 : Logic  Inputs=8  AllPortsSameDT=off  OutDataTypeStr=boolean
  Out1 : Outport
  Out2 : Outport  Port=2
  Out3 : Outport  Port=3
  wires:
  Demux/1 -> NOT1/1
  Demux/2 -> NOT2/1
  Demux/3 -> NOT3/1
  Demux/4 -> NOT4/1
  Demux/5 -> NOT5/1
  Demux/6 -> NOT6/1
  Demux/7 -> NOT7/1
  Demux/8 -> NOT8/1
  Demux1/1 -> NOT1/2
  Demux1/2 -> NOT2/2
  Demux1/3 -> NOT3/2
  Demux1/4 -> NOT4/2
  Demux1/5 -> NOT5/2
  Demux1/6 -> NOT6/2
  Demux1/7 -> NOT7/2
  Demux1/8 -> NOT8/2
  In1/1 -> Demux2/1, Demux/1
  In2/1 -> Demux1/1, Demux3/1
  NOT1/1 -> NOT9/1
  NOT2/1 -> NOT9/2
  NOT3/1 -> NOT9/3
  NOT4/1 -> NOT9/4
  NOT5/1 -> NOT9/5
  NOT6/1 -> NOT9/6
  NOT7/1 -> NOT9/7
  NOT8/1 -> NOT9/8
  NOT9/1 -> Logical Operator25/2, Out2/1
  Logical Operator14/1 -> Logical Operator16/3
  Logical Operator7/1 -> Logical Operator8/1
  Logical Operator13/1 -> Logical Operator15/1, Logical Operator6/3
  Demux3/1 -> Logical Operator9/1
  Demux2/2 -> Logical Operator8/2
  Logical Operator15/1 -> Logical Operator16/1
  Demux2/3 -> Logical Operator13/2
  Logical Operator10/1 -> Logical Operator8/3
  Logical Operator6/1 -> Logical Operator25/1, Out1/1
  Demux2/1 -> Logical Operator5/1
  Demux2/4 -> Logical Operator16/2
  Logical Operator11/1 -> Logical Operator13/3
  Logical Operator16/1 -> Logical Operator24/1, Logical Operator6/4
  Logical Operator9/1 -> Logical Operator5/2
  Demux3/2 -> Logical Operator10/1
  Logical Operator12/1 -> Logical Operator13/1
  Demux3/3 -> Logical Operator11/1
  Demux3/4 -> Logical Operator14/1
  Logical Operator5/1 -> Logical Operator7/1, Logical Operator6/1
  Logical Operator8/1 -> Logical Operator12/1, Logical Operator6/2
  Demux2/5 -> Logical Operator20/1
  Demux3/5 -> Logical Operator23/1
  Logical Operator17/1 -> Logical Operator19/3
  Logical Operator19/1 -> Logical Operator6/8
  Logical Operator1/1 -> Logical Operator22/3
  Logical Operator2/1 -> Logical Operator4/3
  Demux3/8 -> Logical Operator17/1
  Demux3/7 -> Logical Operator2/1
  Demux2/7 -> Logical Operator4/2
  Logical Operator3/1 -> Logical Operator4/1
  Logical Operator21/1 -> Logical Operator22/1
  Logical Operator22/1 -> Logical Operator6/6, Logical Operator3/1
  Demux2/8 -> Logical Operator19/2
  Logical Operator18/1 -> Logical Operator19/1
  Logical Operator20/1 -> Logical Operator6/5, Logical Operator21/1
  Demux3/6 -> Logical Operator1/1
  Logical Operator4/1 -> Logical Operator6/7, Logical Operator18/1
  Demux2/6 -> Logical Operator22/2
  Logical Operator24/1 -> Logical Operator20/2
  Logical Operator23/1 -> Logical Operator20/3
  Logical Operator25/1 -> Out3/1

== system bit32aluhdl/EML_DSP48_Patterns/Comparartor/Comparator3 ==
  In1 : Inport
  In2 : Inport  Port=2
  Demux{,1..3} (4 alike) : Demux  Outputs=8
  Logical Operator{1..3,7,9..12,14..15,17..18,21,23..24} (15 alike) : Logic  Operator=NOT  Inputs=3  AllPortsSameDT=off  OutDataTypeStr=boolean
  Logical Operator{4,8,13,16,19..20,22} (7 alike) : Logic  Inputs=3  AllPortsSameDT=off  OutDataTypeStr=boolean
  Logical Operator25 : Logic  Operator=NOR  AllPortsSameDT=off  OutDataTypeStr=boolean
  Logical Operator5 : Logic  AllPortsSameDT=off  OutDataTypeStr=boolean
  Logical Operator6 : Logic  Operator=OR  Inputs=8  AllPortsSameDT=off  OutDataTypeStr=boolean
  NOT{1..8} (8 alike) : Logic  Operator=NXOR  AllPortsSameDT=off  OutDataTypeStr=boolean
  NOT9 : Logic  Inputs=8  AllPortsSameDT=off  OutDataTypeStr=boolean
  Out1 : Outport
  Out2 : Outport  Port=2
  Out3 : Outport  Port=3
  wires:
  Demux/1 -> NOT1/1
  Demux/2 -> NOT2/1
  Demux/3 -> NOT3/1
  Demux/4 -> NOT4/1
  Demux/5 -> NOT5/1
  Demux/6 -> NOT6/1
  Demux/7 -> NOT7/1
  Demux/8 -> NOT8/1
  Demux1/1 -> NOT1/2
  Demux1/2 -> NOT2/2
  Demux1/3 -> NOT3/2
  Demux1/4 -> NOT4/2
  Demux1/5 -> NOT5/2
  Demux1/6 -> NOT6/2
  Demux1/7 -> NOT7/2
  Demux1/8 -> NOT8/2
  In1/1 -> Demux2/1, Demux/1
  In2/1 -> Demux1/1, Demux3/1
  NOT1/1 -> NOT9/1
  NOT2/1 -> NOT9/2
  NOT3/1 -> NOT9/3
  NOT4/1 -> NOT9/4
  NOT5/1 -> NOT9/5
  NOT6/1 -> NOT9/6
  NOT7/1 -> NOT9/7
  NOT8/1 -> NOT9/8
  NOT9/1 -> Logical Operator25/2, Out2/1
  Logical Operator14/1 -> Logical Operator16/3
  Logical Operator7/1 -> Logical Operator8/1
  Logical Operator13/1 -> Logical Operator15/1, Logical Operator6/3
  Demux3/1 -> Logical Operator9/1
  Demux2/2 -> Logical Operator8/2
  Logical Operator15/1 -> Logical Operator16/1
  Demux2/3 -> Logical Operator13/2
  Logical Operator10/1 -> Logical Operator8/3
  Logical Operator6/1 -> Logical Operator25/1, Out1/1
  Demux2/1 -> Logical Operator5/1
  Demux2/4 -> Logical Operator16/2
  Logical Operator11/1 -> Logical Operator13/3
  Logical Operator16/1 -> Logical Operator24/1, Logical Operator6/4
  Logical Operator9/1 -> Logical Operator5/2
  Demux3/2 -> Logical Operator10/1
  Logical Operator12/1 -> Logical Operator13/1
  Demux3/3 -> Logical Operator11/1
  Demux3/4 -> Logical Operator14/1
  Logical Operator5/1 -> Logical Operator7/1, Logical Operator6/1
  Logical Operator8/1 -> Logical Operator12/1, Logical Operator6/2
  Demux2/5 -> Logical Operator20/1
  Demux3/5 -> Logical Operator23/1
  Logical Operator17/1 -> Logical Operator19/3
  Logical Operator19/1 -> Logical Operator6/8
  Logical Operator1/1 -> Logical Operator22/3
  Logical Operator2/1 -> Logical Operator4/3
  Demux3/8 -> Logical Operator17/1
  Demux3/7 -> Logical Operator2/1
  Demux2/7 -> Logical Operator4/2
  Logical Operator3/1 -> Logical Operator4/1
  Logical Operator21/1 -> Logical Operator22/1
  Logical Operator22/1 -> Logical Operator6/6, Logical Operator3/1
  Demux2/8 -> Logical Operator19/2
  Logical Operator18/1 -> Logical Operator19/1
  Logical Operator20/1 -> Logical Operator6/5, Logical Operator21/1
  Demux3/6 -> Logical Operator1/1
  Logical Operator4/1 -> Logical Operator6/7, Logical Operator18/1
  Demux2/6 -> Logical Operator22/2
  Logical Operator24/1 -> Logical Operator20/2
  Logical Operator23/1 -> Logical Operator20/3
  Logical Operator25/1 -> Out3/1

== system bit32aluhdl/EML_DSP48_Patterns/Decrementer/Subtractor1 ==
  In1 : Inport
  In2 : Inport  Port=2
  Logical Operator2 : Logic  Operator=NOT  AllPortsSameDT=off  OutDataTypeStr=boolean
  Subtractor : Subsystem
  Zeros1 : Constant
  Out1 : Outport
  Out2 : Outport  Port=2
  wires:
  In2/1 -> Logical Operator2/1
  Subtractor/1(Out1) -> Out1/1
  In1/1 -> Subtractor/1(In1)
  Subtractor/2(Out2) -> Out2/1
  Logical Operator2/1 -> Subtractor/3(In3)
  Zeros1/1 -> Subtractor/2(In2)

== system bit32aluhdl/EML_DSP48_Patterns/Decrementer1/Subtractor1 ==
  In1 : Inport
  In2 : Inport  Port=2
  Logical Operator2 : Logic  Operator=NOT  AllPortsSameDT=off  OutDataTypeStr=boolean
  Subtractor : Subsystem
  Zeros1 : Constant
  Out1 : Outport
  Out2 : Outport  Port=2
  wires:
  In2/1 -> Logical Operator2/1
  Subtractor/1(Out1) -> Out1/1
  In1/1 -> Subtractor/1(In1)
  Subtractor/2(Out2) -> Out2/1
  Logical Operator2/1 -> Subtractor/3(In3)
  Zeros1/1 -> Subtractor/2(In2)

== system bit32aluhdl/EML_DSP48_Patterns/Incrementer/Incrementer ==
  In1 : Inport
  In2 : Inport  Port=2
  Subsystem : Subsystem
  Zeros1 : Constant  Value=0
  Out1 : Outport
  Out2 : Outport  Port=2
  wires:
  Subsystem/2(Out2) -> Out2/1
  In2/1 -> Subsystem/3(In3)
  Zeros1/1 -> Subsystem/2(In2)
  In1/1 -> Subsystem/1(In1)
  Subsystem/1(Out1) -> Out1/1

== system bit32aluhdl/EML_DSP48_Patterns/Incrementer1/Incrementer ==
  In1 : Inport
  In2 : Inport  Port=2
  Subsystem : Subsystem
  Zeros1 : Constant  Value=0
  Out1 : Outport
  Out2 : Outport  Port=2
  wires:
  Subsystem/2(Out2) -> Out2/1
  In2/1 -> Subsystem/3(In3)
  Zeros1/1 -> Subsystem/2(In2)
  In1/1 -> Subsystem/1(In1)
  Subsystem/1(Out1) -> Out1/1

== system bit32aluhdl/EML_DSP48_Patterns/Multiplier/Subsystem ==
  In1 : Inport
  In2 : Inport  Port=2
  In3 : Inport  Port=3
  Demux : Demux  Outputs=2
  Demux1 : Demux  Outputs=2
  Mux : Mux  Inputs=2
  Subsystem1 : Subsystem
  Subsystem2 : Subsystem
  Out1 : Outport
  Out2 : Outport  Port=2
  wires:
  Mux/1 -> Out2/1
  In3/1 -> Demux1/1
  Subsystem2/2(Out2) -> Mux/2
  In1/1 -> Demux/1
  Subsystem2/1(Out1) -> Subsystem1/2(In2)
  Subsystem1/2(Out2) -> Mux/1
  Demux1/2 -> Subsystem2/3(In3)
  In2/1 -> Subsystem2/2(In2)
  Demux/2 -> Subsystem2/1(In1)
  Subsystem1/1(Out1) -> Out1/1
  Demux1/1 -> Subsystem1/3(In3)
  Demux/1 -> Subsystem1/1(In1)

== system bit32aluhdl/EML_DSP48_Patterns/Multiplier/Subsystem1 ==
  In1 : Inport
  In2 : Inport  Port=2
  Constant17 : Constant  Value=0
  Demux : Demux  Outputs=16
  Demux1 : Demux  Outputs=16
  Display1 : Display
  Logical Operator : Logic  Operator=XOR  AllPortsSameDT=off  OutDataTypeStr=boolean
  Logical Operator1 : Logic  AllPortsSameDT=off  OutDataTypeStr=boolean
  Mux : Mux  Inputs=16
  Mux1 : Mux  Inputs=16
  Subsystem : Subsystem
  Subsystem1 : Subsystem
  Subsystem2 : Subsystem
  Subsystem3 : Subsystem
  Subsystem4 : Subsystem
  Subsystem5 : Subsystem
  Subsystem6 : Subsystem
  Out1 : Outport
  Out2 : Outport  Port=2
  wires:
  Subsystem3/11(Out11) -> Subsystem/27(In27)
  Subsystem5/16(Out16) -> Mux1/7
  Subsystem/16(Out16) -> Subsystem5/15(In23)
  Subsystem5/7(Out7) -> Subsystem6/30(In30)
  Subsystem2/14(Out14) -> Subsystem/14(In22)
  Subsystem4/9(Out9) -> Mux1/9
  Subsystem5/11(Out11) -> Mux1/2
  Subsystem2/15(Out15) -> Subsystem/15(In23)
  Subsystem3/16(Out16) -> Subsystem/32(In32)
  Subsystem3/6(Out6) -> Subsystem/22(In14)
  Subsystem6/10(Out10) -> Mux/9
  Subsystem5/2(Out2) -> Subsystem6/25(In25)
  Subsystem4/7(Out7) -> Subsystem5/31(In31)
  Subsystem2/11(Out11) -> Subsystem/11(In19)
  Subsystem3/9(Out9) -> Subsystem/25(In25)
  Subsystem1/2(Out2) -> Subsystem6/2(In2)
  Subsystem1/3(Out3) -> Subsystem6/3(In3)
  Subsystem/17(Out17) -> Subsystem5/16(In24)
  Subsystem/4(Out4) -> Subsystem5/3(In3)
  Subsystem3/8(Out8) -> Subsystem/24(In16)
  Subsystem/11(Out11) -> Subsystem5/10(In18)
  Logical Operator1/1 -> Subsystem6/23(In15)
  Subsystem3/2(Out2) -> Subsystem/18(In10)
  Subsystem1/13(Out13) -> Subsystem6/13(14)
  Subsystem4/4(Out4) -> Subsystem5/28(In28)
  Subsystem5/17(Out17) -> Mux1/8
  Subsystem5/5(Out5) -> Subsystem6/28(In28)
  Subsystem1/8(Out8) -> Subsystem6/8(In8)
  Subsystem2/3(Out3) -> Subsystem/3(In3)
  Subsystem5/6(Out6) -> Subsystem6/29(In29)
  Subsystem/2(Out2) -> Subsystem5/1(In1)
  Subsystem4/1(Out1) -> Subsystem5/25(In25)
  Subsystem1/7(Out7) -> Subsystem6/7(In7)
  Subsystem5/9(Out9) -> Subsystem6/32(In32)
  Subsystem6/8(Out8) -> Mux/7
  Subsystem1/5(Out5) -> Subsystem6/5(In5)
  Subsystem6/11(Out11) -> Mux/10
  Subsystem1/6(Out6) -> Subsystem6/6(In6)
  Subsystem/7(Out7) -> Subsystem5/6(In6)
  Subsystem2/16(Out16) -> Subsystem/16(In24)
  Demux/7 -> Subsystem2/7(In7), Subsystem1/7(In7)
  Demux1/14 -> Subsystem4/14(In14), Subsystem2/14(In14)
  Demux/16 -> Subsystem4/8(In8), Subsystem3/8(In8)
  Subsystem2/1(Out1) -> Subsystem/1(In1)
  Subsystem5/15(Out15) -> Mux1/6
  Subsystem4/16(Out16) -> Mux1/16
  Subsystem3/4(Out4) -> Subsystem/20(In12)
  Subsystem/1(Out1) -> Logical Operator1/2, Logical Operator/2
  Subsystem1/4(Out4) -> Subsystem6/4(In4)
  Subsystem4/11(Out11) -> Mux1/11
  Demux/1 -> Subsystem1/1(In1), Subsystem2/1(In1)
  Subsystem3/10(Out10) -> Subsystem/26(In26)
  Subsystem6/2(Out2) -> Mux/1
  Subsystem/9(Out9) -> Subsystem5/8(In8)
  Demux1/3 -> Subsystem3/11(In11), Subsystem1/11(In11)
  Demux1/7 -> Subsystem3/15(In15), Subsystem1/15(In15)
  Subsystem/5(Out5) -> Subsystem5/4(In4)
  Mux/1 -> Out1/1
  Subsystem5/10(Out10) -> Mux1/1
  Subsystem1/12(Out12) -> Subsystem6/12(In20)
  Subsystem2/6(Out6) -> Subsystem/6(In6)
  Demux/13 -> Subsystem4/5(In5), Subsystem3/5(In5)
  Demux/10 -> Subsystem4/2(In2), Subsystem3/2(In2)
  Demux/11 -> Subsystem4/3(In3), Subsystem3/3(In3)
  Subsystem1/11(Out11) -> Subsystem6/11(In19)
  Subsystem6/17(Out17) -> Mux/16
  Demux/9 -> Subsystem4/1(In1), Subsystem3/1(In1)
  Subsystem4/15(Out15) -> Mux1/15
  Subsystem5/8(Out8) -> Subsystem6/31(In31)
  Demux1/1 -> Subsystem1/9(In9), Subsystem3/9(In9)
  Demux1/2 -> Subsystem3/10(In10), Subsystem1/10(In10)
  Demux/8 -> Subsystem2/8(In8), Subsystem1/8(In8)
  Demux/14 -> Subsystem4/6(In6), Subsystem3/6(In6)
  Subsystem1/15(Out15) -> Subsystem6/15(In23)
  Demux1/9 -> Subsystem2/9(In9), Subsystem4/9(In9)
  Subsystem5/14(Out14) -> Mux1/5
  Demux/6 -> Subsystem1/6(In6), Subsystem2/6(In6)
  Subsystem2/7(Out7) -> Subsystem/7(In7)
  Subsystem2/4(Out4) -> Subsystem/4(In4)
  Demux1/5 -> Subsystem3/13(In13), Subsystem1/13(In13)
  Subsystem/8(Out8) -> Subsystem5/7(In7)
  Logical Operator/1 -> Subsystem6/24(In16)
  Demux1/12 -> Subsystem2/12(In12), Subsystem4/12(In12)
  Subsystem2/9(Out9) -> Subsystem/9(In17)
  Subsystem5/13(Out13) -> Mux1/4
  Subsystem5/3(Out3) -> Subsystem6/26(In26)
  Demux1/8 -> Subsystem1/16(In16), Subsystem3/16(In16)
  Subsystem4/14(Out14) -> Mux1/14
  Constant17/1 -> Subsystem5/24(In16), Subsystem5/23(In15), Subsystem5/22(In14), Subsystem5/21(In13), Subsystem5/20(In12), Subsystem5/19(In11), Subsystem5/18(In10), Subsystem5/17(In9), Subsystem6/17(In9), Subsystem6/18(In10), Subsystem6/20(In12), Subsystem6/21(In13), Subsystem6/22(In14), Subsystem6/19(In11)
  Subsystem3/13(Out13) -> Subsystem/29(In29)
  Subsystem1/16(Out16) -> Subsystem6/16(In24)
  Subsystem/15(Out15) -> Subsystem5/14(In22)
  Demux1/13 -> Subsystem2/13(In13), Subsystem4/13(In13)
  Subsystem/12(Out12) -> Subsystem5/11(In19)
  Demux1/16 -> Subsystem2/16(In16), Subsystem4/16(In16)
  Subsystem5/12(Out12) -> Mux1/3
  Subsystem3/15(Out15) -> Subsystem/31(In31)
  Subsystem6/9(Out9) -> Mux/8
  Demux/5 -> Subsystem1/5(In5), Subsystem2/5(In5)
  Subsystem6/4(Out4) -> Mux/3
  Subsystem6/3(Out3) -> Mux/2
  Subsystem4/13(Out13) -> Mux1/13
  Demux1/6 -> Subsystem3/14(In14), Subsystem1/14(In14)
  Subsystem/6(Out6) -> Subsystem5/5(In5)
  Subsystem/13(Out13) -> Subsystem5/12(In20)
  Subsystem6/13(Out13) -> Mux/12
  Subsystem6/12(Out12) -> Mux/11
  Subsystem4/10(Out10) -> Mux1/10
  Subsystem3/5(Out5) -> Subsystem/21(In13)
  Subsystem/10(Out10) -> Subsystem5/9(In17)
  Subsystem2/12(Out12) -> Subsystem/12(In20)
  Subsystem5/1(Out1) -> Logical Operator/1, Logical Operator1/1
  Subsystem6/5(Out5) -> Mux/4
  Subsystem3/1(Out1) -> Subsystem/17(In9)
  Subsystem4/8(Out8) -> Subsystem5/32(In32)
  Subsystem3/12(Out12) -> Subsystem/28(In28)
  Subsystem6/1(Out1) -> Display1/1
  Subsystem4/6(Out6) -> Subsystem5/30(In30)
  Subsystem2/2(Out2) -> Subsystem/2(In2)
  Subsystem2/10(Out10) -> Subsystem/10(In18)
  Subsystem4/5(Out5) -> Subsystem5/29(In29)
  Subsystem2/13(Out13) -> Subsystem/13(14)
  Subsystem1/1(Out1) -> Subsystem6/1(In1)
  Subsystem6/7(Out7) -> Mux/6
  Subsystem6/14(Out14) -> Mux/13
  Subsystem5/4(Out4) -> Subsystem6/27(In27)
  Subsystem2/8(Out8) -> Subsystem/8(In8)
  Subsystem/14(Out14) -> Subsystem5/13(14)
  Subsystem6/16(Out16) -> Mux/15
  Demux/4 -> Subsystem2/4(In4), Subsystem1/4(In4)
  Subsystem1/10(Out10) -> Subsystem6/10(In18)
  Demux/12 -> Subsystem4/4(In4), Subsystem3/4(In4)
  Subsystem3/14(Out14) -> Subsystem/30(In30)
  Subsystem2/5(Out5) -> Subsystem/5(In5)
  Demux1/10 -> Subsystem2/10(In10), Subsystem4/10(In10)
  Demux/2 -> Subsystem1/2(In2), Subsystem2/2(In2)
  Subsystem6/6(Out6) -> Mux/5
  Subsystem/3(Out3) -> Subsystem5/2(In2)
  Subsystem4/12(Out12) -> Mux1/12
  Demux1/4 -> Subsystem1/12(In12), Subsystem3/12(In12)
  Demux/15 -> Subsystem4/7(In7), Subsystem3/7(In7)
  Subsystem1/14(Out14) -> Subsystem6/14(In22)
  Subsystem3/3(Out3) -> Subsystem/19(In11)
  Subsystem6/15(Out15) -> Mux/14
  Subsystem1/9(Out9) -> Subsystem6/9(In17)
  Demux1/11 -> Subsystem2/11(In11), Subsystem4/11(In11)
  Subsystem4/2(Out2) -> Subsystem5/26(In26)
  Demux/3 -> Subsystem1/3(In3), Subsystem2/3(In3)
  Subsystem4/3(Out3) -> Subsystem5/27(In27)
  Subsystem3/7(Out7) -> Subsystem/23(In15)
  Demux1/15 -> Subsystem2/15(In15), Subsystem4/15(In15)
  In1/1 -> Demux/1
  In2/1 -> Demux1/1
  Mux1/1 -> Out2/1
